simulink model "lab6csim"  (R2022b)
settings: Solver=FixedStepAuto  StartTime=0.0  StopTime=1.9*10  FixedStep=10/(1024*2^5)  RelTol=1e-3
undefined symbols (not defined in the file or in its folder): DiscIntNeverNeededParam, lutdata, lutix
libraries: dsparch4 x1
settings Model: Creator=andjog  LastModifiedBy=andjog

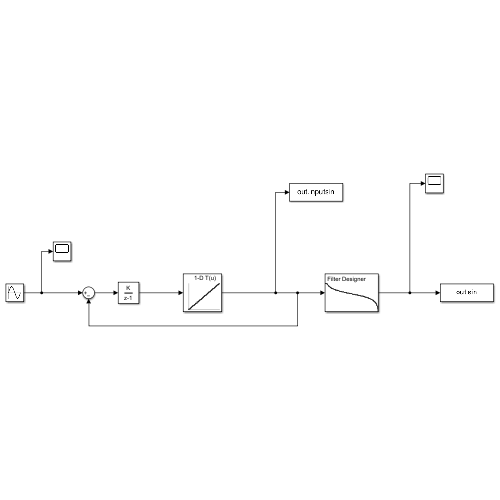
[thumbnail: Simulink's stored preview of the top-level diagram]
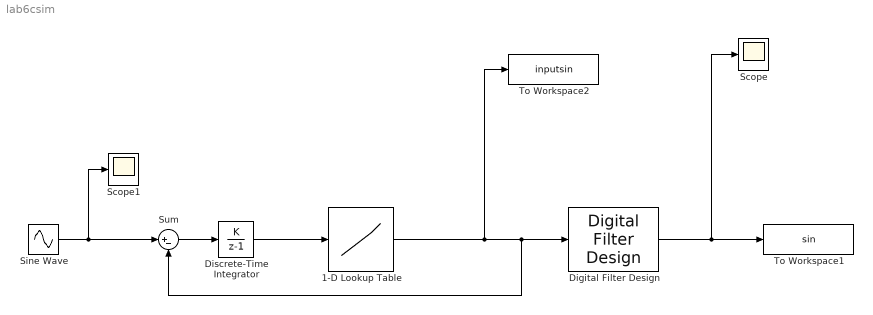
== system lab6csim ==
  1-D Lookup Table : Lookup_n-D  NumberOfTableDimensions=1  BreakpointsForDimension1=lutix(2^7)  Table=lutdata(2^7)  InternalRulePriority=Speed  RndMeth=Simplest
  Digital Filter Design : dsparch4/Digital Filter Design  mwdsp_browser_bugfix_var=off
  Discrete-Time Integrator : DiscreteIntegrator  IntegratorMethod=Accumulation: Forward Euler  SampleTime=-1  ICPrevOutput=DiscIntNeverNeededParam  ICPrevScaledInput=DiscIntNeverNeededParam
  Scope : Scope
  Scope1 : Scope
  Sine Wave : Sin  Frequency=pi  SampleTime=0
  Sum : Sum  Inputs=|+-
  To Workspace1 : ToWorkspace  VariableName=sin  SaveFormat=Structure With Time  SampleTime=-1
  To Workspace2 : ToWorkspace  VariableName=inputsin  SaveFormat=Structure With Time  SampleTime=-1
  wires:
  Sine Wave/1 -> Scope1/1, Sum/1
  1-D Lookup Table/1 -> Digital Filter Design/1, Sum/2, To Workspace2/1
  Sum/1 -> Discrete-Time Integrator/1
  Discrete-Time Integrator/1 -> 1-D Lookup Table/1
  Digital Filter Design/1 -> Scope/1, To Workspace1/1
